simulink model "zero_crossing_detection"  (R2021a)
settings: Solver=VariableStepAuto  StartTime=0.0  StopTime=10.0  RelTol=1e-3
libraries: dspswit3 x1, dspsigops x1
settings Model: Creator=Acer  LastModifiedBy=Acer

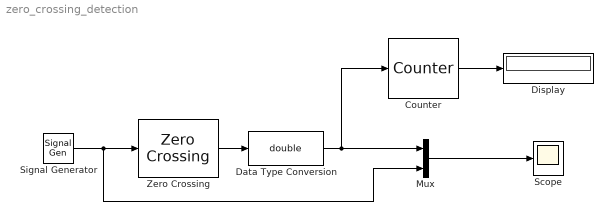
== system zero_crossing_detection ==
  Counter : dspswit3/Counter  Direction=Up  CountEvent=Rising edge  CounterSize=8 bits  MaxCount=255  InitialCount=0  Output=Count  HitValue=32  ResetInput=off  SamplesPerFrame=1  Ts=1  CntDtype=double  HitDtype=Logical
  Data Type Conversion : DataTypeConversion  OutDataTypeStr=double
  Display : Display
  Mux : Mux  Inputs=2
  Scope : Scope
  Signal Generator : SignalGenerator  WaveForm=random  Units=rad/sec
  Zero Crossing : dspsigops/Zero Crossing  InputProcessing=Columns as channels (frame based)
      settings: SourceProductBaseCode=DS
  wires:
  Data Type Conversion/1 -> Mux/1, Counter/1
  Signal Generator/1 -> Mux/2, Zero Crossing/1
  Zero Crossing/1 -> Data Type Conversion/1
  Counter/1 -> Display/1
  Mux/1 -> Scope/1
